simulink model "MultipleAgentsChoice_NoVR"  (Simulink 7.5)
settings: Solver=ode45  StartTime=0.0  StopTime=1000  RelTol=1e-4  AbsTol=1e-4
libraries: simulink x64
(part 4 of 6)

== system MultipleAgentsChoice_NoVR/StatePropagation/SatelliteControlAccel/Agent Body3/Actual Thruster response/Zthruster1 ==
  note: NB:-Agent has no knowledge of red blocks
      |             -Blue blocks prescribed by agent
  note: Tank pressure and thruster selection: must declare number of thrusters
  FeedPressure : Inport  OutDataType=sfix(16)  OutScaling=2^0
  ForceRequest : Inport  Port=2  OutDataType=sfix(16)  OutScaling=2^0
  Data : Inport  Port=3  OutDataType=sfix(16)  OutScaling=2^0
  Reliability : Inport  Port=4  OutDataType=sfix(16)  OutScaling=2^0
  BrokenLine : Inport  Port=5  OutDataType=sfix(16)  OutScaling=2^0
  Bus Creator2 : BusCreator  Inputs=3
  Bus Selector : BusSelector  OutputSignals=ZValves,ZSwitch
  Constant : Constant  OutDataType=sfix(16)  OutScaling=2^0
  Constant1 : Constant  Value=0  OutDataType=sfix(16)  OutScaling=2^0
  Switch : Switch  Criteria=u2 ~= 0
  Thruster1 : Subsystem
  ZData : Outport  OutDataType=sfix(16)  OutScaling=2^0
  Zforces : Outport  Port=2  OutDataType=sfix(16)  OutScaling=2^0
  Activitydata : Outport  Port=3  OutDataType=sfix(16)  OutScaling=2^0
  wires:
  ForceRequest/1 -> Thruster1/4(ForceRequest)  "Zforces"
  Thruster1/1(L1Vent) -> Bus Creator2/1  "L1Vent"
  Thruster1/2(L2Vent) -> Bus Creator2/2  "L2Vent"
  FeedPressure/1 -> Thruster1/2(FeedPressure)
  Constant/1 -> Switch/1
  Constant1/1 -> Switch/3
  Thruster1/4(thrusterData) -> ZData/1  "A3TZ"
  Data/1 -> Bus Selector/1
  Bus Selector/1 -> Thruster1/1(ValveAssign)  "<ZValves>"
  Bus Selector/2 -> Thruster1/3(MainSwitch)  "<ZSwitch>"
  Thruster1/3(Forces) -> Zforces/1, Switch/2
  Switch/1 -> Bus Creator2/3  "Active1"
  Bus Creator2/1 -> Activitydata/1
  Reliability/1 -> Thruster1/5(Reliability)
  BrokenLine/1 -> Thruster1/6(BrokenLine)

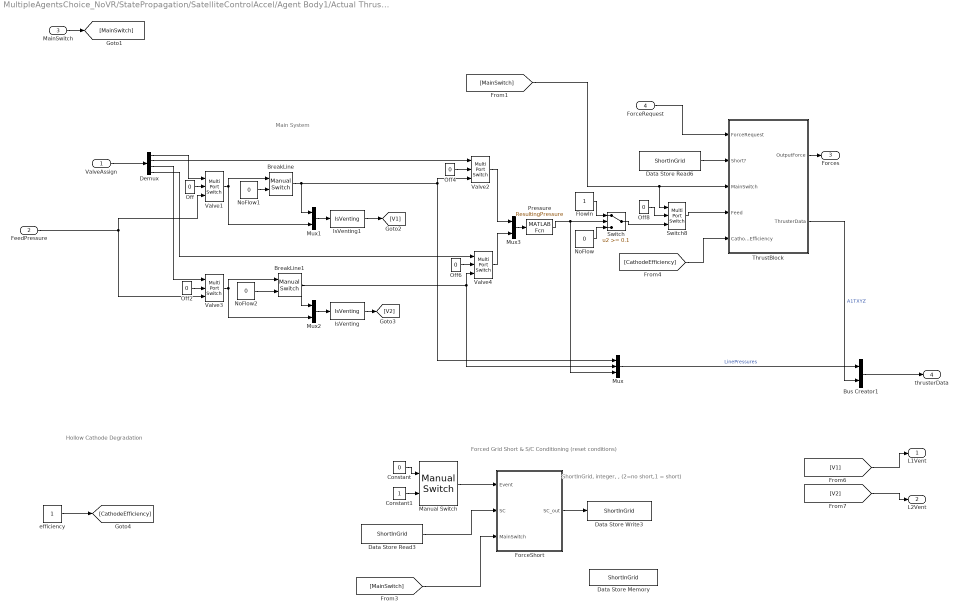
== system MultipleAgentsChoice_NoVR/StatePropagation/SatelliteControlAccel/Agent Body1/Actual Thruster response/XYZthruster/Thruster1 ==
  note: Forced Grid Short & S/C Conditioning (reset conditions)
  note: ShortInGrid, integer, , (2=no short,1 = short)
  note: Hollow Cathode Degradation
  note: Main System
  ValveAssign : Inport  OutDataType=sfix(16)  OutScaling=2^0
  FeedPressure : Inport  Port=2  OutDataType=sfix(16)  OutScaling=2^0
  MainSwitch : Inport  Port=3  OutDataType=sfix(16)  OutScaling=2^0
  ForceRequest : Inport  Port=4  OutDataType=sfix(16)  OutScaling=2^0
  BreakLine : simulink/Signal Routing/Manual Switch  SystemSampleTime=-1  sw=1  action=0  varsize=off
  BreakLine1 : simulink/Signal Routing/Manual Switch  SystemSampleTime=-1  sw=1  action=0  varsize=off
  Bus Creator1 : BusCreator  Inputs=2
  Constant : Constant  Value=0  OutDataType=sfix(16)  OutScaling=2^0
  Constant1 : Constant  OutDataType=sfix(16)  OutScaling=2^0
  Data Store Memory : DataStoreMemory  DataStoreName=ShortInGrid  ReadBeforeWriteMsg=warning  WriteAfterWriteMsg=warning  WriteAfterReadMsg=warning  InitialValue=2  OutDataType=sfix(16)  OutScaling=2^0
  Data Store Read3 : DataStoreRead  DataStoreName=ShortInGrid  SampleTime=0
  Data Store Read6 : DataStoreRead  DataStoreName=ShortInGrid  SampleTime=0
  Data Store Write3 : DataStoreWrite  DataStoreName=ShortInGrid  SampleTime=-1
  Demux : Demux
  FlowIn : Constant  OutDataType=sfix(16)  OutScaling=2^0
  ForceShort : Subsystem
  IsVenting : MATLABFcn  MATLABFcn=IsVenting  OutputDimensions=1
  IsVenting1 : MATLABFcn  MATLABFcn=IsVenting  OutputDimensions=1
  Manual Switch : simulink/Signal Routing/Manual Switch  SystemSampleTime=-1  sw=1  action=0  varsize=off
  Mux : Mux  Inputs=3
  Mux1 : Mux  Inputs=2
  Mux2 : Mux  Inputs=2
  Mux3 : Mux  Inputs=2
  NoFlow : Constant  Value=0  OutDataType=sfix(16)  OutScaling=2^0
  NoFlow1 : Constant  Value=0  OutDataType=sfix(16)  OutScaling=2^0
  NoFlow2 : Constant  Value=0  OutDataType=sfix(16)  OutScaling=2^0
  Off{,2,4,6,8} (5 alike) : Constant  Value=0  OutDataType=sfix(16)  OutScaling=2^0
  Pressure : MATLABFcn  MATLABFcn=ResultingPressure
  Switch : Switch  Threshold=0.1
  Switch8 : MultiPortSwitch  Inputs=2  zeroidx=off
  ThrustBlock : Subsystem
  Valve{1..4} (4 alike) : MultiPortSwitch  Inputs=2  zeroidx=off
  efficiency : Constant  OutDataType=sfix(16)  OutScaling=2^0
  L1Vent : Outport  OutDataType=sfix(16)  OutScaling=2^0
  L2Vent : Outport  Port=2  OutDataType=sfix(16)  OutScaling=2^0
  Forces : Outport  Port=3  OutDataType=sfix(16)  OutScaling=2^0
  thrusterData : Outport  Port=4  OutDataType=sfix(16)  OutScaling=2^0
  wires:
  ForceShort/1(SC_out) -> Data Store Write3/1
  Constant/1 -> Manual Switch/1
  Constant1/1 -> Manual Switch/2
  Manual Switch/1 -> ForceShort/1(Event)
  Data Store Read3/1 -> ForceShort/2(SC)
  [MainSwitch] -> ForceShort/3(MainSwitch)
  efficiency/1 -> [CathodeEfficiency]
  Valve1/1 -> BreakLine/1, Mux1/2
  Valve2/1 -> Mux3/1
  Mux3/1 -> Pressure/1
  BreakLine/1 -> Mux1/1, Valve2/3, Mux/1
  FlowIn/1 -> Switch/1
  NoFlow/1 -> Switch/3
  Switch8/1 -> ThrustBlock/4(Feed)
  Data Store Read6/1 -> ThrustBlock/2(Short?)
  ValveAssign/1 -> Demux/1
  Demux/1 -> Valve1/1
  Demux/2 -> Valve2/1
  Demux/3 -> Valve3/1
  Demux/4 -> Valve4/1
  ThrustBlock/2(ThrusterData) -> Bus Creator1/2  "A1TXYZ"
  ThrustBlock/1(OutputForce) -> Forces/1
  NoFlow1/1 -> BreakLine/2
  Off/1 -> Valve1/2
  Off4/1 -> Valve2/2
  Off2/1 -> Valve3/2
  Off6/1 -> Valve4/2
  Off8/1 -> Switch8/2
  Switch/1 -> Switch8/3
  Mux/1 -> Bus Creator1/1  "LinePressures"
  NoFlow2/1 -> BreakLine1/2
  Valve3/1 -> BreakLine1/1, Mux2/2
  BreakLine1/1 -> Mux2/1, Valve4/3, Mux/2
  [CathodeEfficiency] -> ThrustBlock/5(CathodeEfficiency)
  ForceRequest/1 -> ThrustBlock/1(ForceRequest)
  Bus Creator1/1 -> thrusterData/1
  Mux1/1 -> IsVenting1/1
  Mux2/1 -> IsVenting/1
  Pressure/1 -> Switch/2, Mux/3
  IsVenting1/1 -> [V1]
  IsVenting/1 -> [V2]
  FeedPressure/1 -> Valve1/3, Valve3/3
  MainSwitch/1 -> [MainSwitch]
  Valve4/1 -> Mux3/2
  [MainSwitch] -> ThrustBlock/3(MainSwitch), Switch8/1
  [V1] -> L1Vent/1
  [V2] -> L2Vent/1

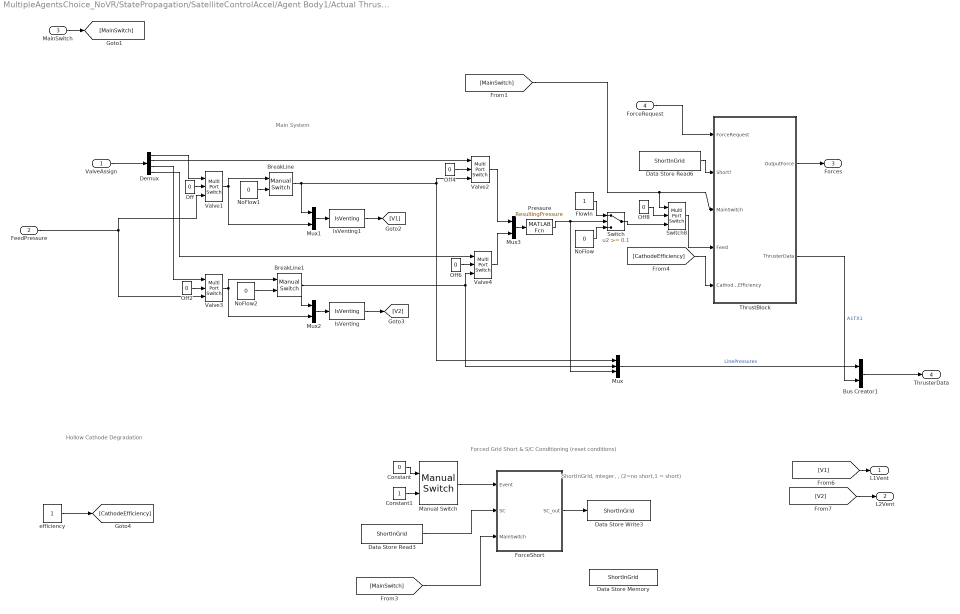
== system MultipleAgentsChoice_NoVR/StatePropagation/SatelliteControlAccel/Agent Body1/Actual Thruster response/Xthruster/Thruster1 ==
  note: Main System
  note: Hollow Cathode Degradation
  note: ShortInGrid, integer, , (2=no short,1 = short)
  note: Forced Grid Short & S/C Conditioning (reset conditions)
  ValveAssign : Inport  OutDataType=sfix(16)  OutScaling=2^0
  FeedPressure : Inport  Port=2  OutDataType=sfix(16)  OutScaling=2^0
  MainSwitch : Inport  Port=3  OutDataType=sfix(16)  OutScaling=2^0
  ForceRequest : Inport  Port=4  OutDataType=sfix(16)  OutScaling=2^0
  BreakLine : simulink/Signal Routing/Manual Switch  SystemSampleTime=-1  sw=1  action=0  varsize=off
  BreakLine1 : simulink/Signal Routing/Manual Switch  SystemSampleTime=-1  sw=1  action=0  varsize=off
  Bus Creator1 : BusCreator  Inputs=2
  Constant : Constant  Value=0  OutDataType=sfix(16)  OutScaling=2^0
  Constant1 : Constant  OutDataType=sfix(16)  OutScaling=2^0
  Data Store Memory : DataStoreMemory  DataStoreName=ShortInGrid  ReadBeforeWriteMsg=warning  WriteAfterWriteMsg=warning  WriteAfterReadMsg=warning  InitialValue=2  OutDataType=sfix(16)  OutScaling=2^0
  Data Store Read3 : DataStoreRead  DataStoreName=ShortInGrid  SampleTime=0
  Data Store Read6 : DataStoreRead  DataStoreName=ShortInGrid  SampleTime=0
  Data Store Write3 : DataStoreWrite  DataStoreName=ShortInGrid  SampleTime=-1
  Demux : Demux
  FlowIn : Constant  OutDataType=sfix(16)  OutScaling=2^0
  ForceShort : Subsystem
  IsVenting : MATLABFcn  MATLABFcn=IsVenting  OutputDimensions=1
  IsVenting1 : MATLABFcn  MATLABFcn=IsVenting  OutputDimensions=1
  Manual Switch : simulink/Signal Routing/Manual Switch  SystemSampleTime=-1  sw=1  action=0  varsize=off
  Mux : Mux  Inputs=3
  Mux1 : Mux  Inputs=2
  Mux2 : Mux  Inputs=2
  Mux3 : Mux  Inputs=2
  NoFlow : Constant  Value=0  OutDataType=sfix(16)  OutScaling=2^0
  NoFlow1 : Constant  Value=0  OutDataType=sfix(16)  OutScaling=2^0
  NoFlow2 : Constant  Value=0  OutDataType=sfix(16)  OutScaling=2^0
  Off{,2,4,6,8} (5 alike) : Constant  Value=0  OutDataType=sfix(16)  OutScaling=2^0
  Pressure : MATLABFcn  MATLABFcn=ResultingPressure
  Switch : Switch  Threshold=0.1
  Switch8 : MultiPortSwitch  Inputs=2  zeroidx=off
  ThrustBlock : Subsystem
  Valve{1..4} (4 alike) : MultiPortSwitch  Inputs=2  zeroidx=off
  efficiency : Constant  OutDataType=sfix(16)  OutScaling=2^0
  L1Vent : Outport  OutDataType=sfix(16)  OutScaling=2^0
  L2Vent : Outport  Port=2  OutDataType=sfix(16)  OutScaling=2^0
  Forces : Outport  Port=3  OutDataType=sfix(16)  OutScaling=2^0
  ThrusterData : Outport  Port=4  OutDataType=sfix(16)  OutScaling=2^0
  wires:
  [MainSwitch] -> Switch8/1, ThrustBlock/3(MainSwitch)
  Valve4/1 -> Mux3/2
  MainSwitch/1 -> [MainSwitch]
  FeedPressure/1 -> Valve3/3, Valve1/3
  IsVenting/1 -> [V2]
  IsVenting1/1 -> [V1]
  Pressure/1 -> Mux/3, Switch/2
  Mux2/1 -> IsVenting/1
  Mux1/1 -> IsVenting1/1
  Bus Creator1/1 -> ThrusterData/1
  ForceRequest/1 -> ThrustBlock/1(ForceRequest)
  [CathodeEfficiency] -> ThrustBlock/5(CathodeEfficiency)
  BreakLine1/1 -> Mux/2, Valve4/3, Mux2/1
  Valve3/1 -> Mux2/2, BreakLine1/1
  NoFlow2/1 -> BreakLine1/2
  Mux/1 -> Bus Creator1/1  "LinePressures"
  Switch/1 -> Switch8/3
  Off8/1 -> Switch8/2
  Off6/1 -> Valve4/2
  Off2/1 -> Valve3/2
  Off4/1 -> Valve2/2
  Off/1 -> Valve1/2
  NoFlow1/1 -> BreakLine/2
  ThrustBlock/1(OutputForce) -> Forces/1
  ThrustBlock/2(ThrusterData) -> Bus Creator1/2  "A1TX1"
  Demux/4 -> Valve4/1
  Demux/3 -> Valve3/1
  Demux/2 -> Valve2/1
  Demux/1 -> Valve1/1
  ValveAssign/1 -> Demux/1
  Data Store Read6/1 -> ThrustBlock/2(Short?)
  Switch8/1 -> ThrustBlock/4(Feed)
  NoFlow/1 -> Switch/3
  FlowIn/1 -> Switch/1
  BreakLine/1 -> Mux/1, Valve2/3, Mux1/1
  Mux3/1 -> Pressure/1
  Valve2/1 -> Mux3/1
  Valve1/1 -> Mux1/2, BreakLine/1
  efficiency/1 -> [CathodeEfficiency]
  [MainSwitch] -> ForceShort/3(MainSwitch)
  Data Store Read3/1 -> ForceShort/2(SC)
  Manual Switch/1 -> ForceShort/1(Event)
  Constant1/1 -> Manual Switch/2
  Constant/1 -> Manual Switch/1
  ForceShort/1(SC_out) -> Data Store Write3/1
  [V1] -> L1Vent/1
  [V2] -> L2Vent/1

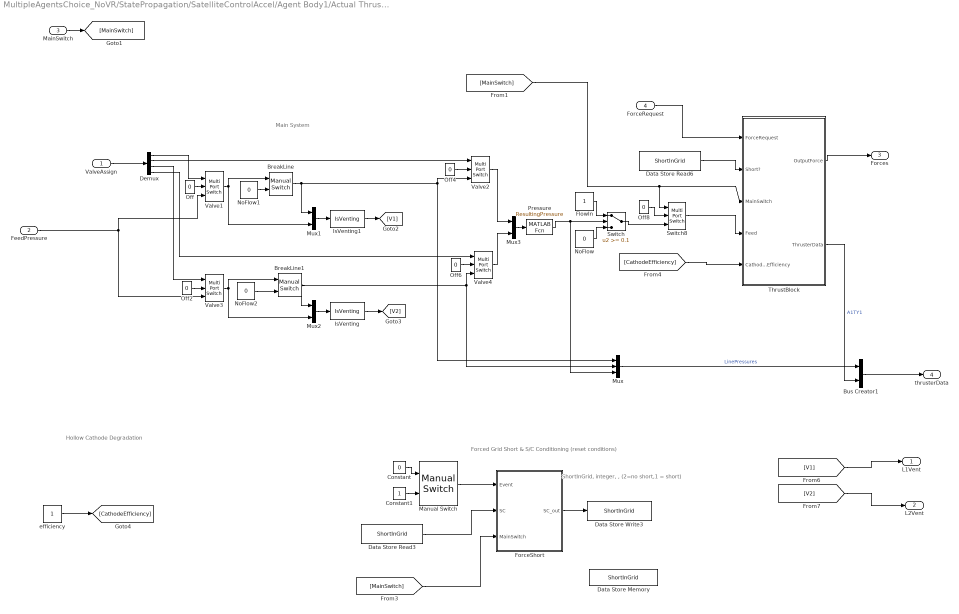
== system MultipleAgentsChoice_NoVR/StatePropagation/SatelliteControlAccel/Agent Body1/Actual Thruster response/Ythruster1/Thruster1 ==
  note: Forced Grid Short & S/C Conditioning (reset conditions)
  note: ShortInGrid, integer, , (2=no short,1 = short)
  note: Hollow Cathode Degradation
  note: Main System
  ValveAssign : Inport  OutDataType=sfix(16)  OutScaling=2^0
  FeedPressure : Inport  Port=2  OutDataType=sfix(16)  OutScaling=2^0
  MainSwitch : Inport  Port=3  OutDataType=sfix(16)  OutScaling=2^0
  ForceRequest : Inport  Port=4  OutDataType=sfix(16)  OutScaling=2^0
  BreakLine : simulink/Signal Routing/Manual Switch  SystemSampleTime=-1  sw=1  action=0  varsize=off
  BreakLine1 : simulink/Signal Routing/Manual Switch  SystemSampleTime=-1  sw=1  action=0  varsize=off
  Bus Creator1 : BusCreator  Inputs=2
  Constant : Constant  Value=0  OutDataType=sfix(16)  OutScaling=2^0
  Constant1 : Constant  OutDataType=sfix(16)  OutScaling=2^0
  Data Store Memory : DataStoreMemory  DataStoreName=ShortInGrid  ReadBeforeWriteMsg=warning  WriteAfterWriteMsg=warning  WriteAfterReadMsg=warning  InitialValue=2  OutDataType=sfix(16)  OutScaling=2^0
  Data Store Read3 : DataStoreRead  DataStoreName=ShortInGrid  SampleTime=0
  Data Store Read6 : DataStoreRead  DataStoreName=ShortInGrid  SampleTime=0
  Data Store Write3 : DataStoreWrite  DataStoreName=ShortInGrid  SampleTime=-1
  Demux : Demux
  FlowIn : Constant  OutDataType=sfix(16)  OutScaling=2^0
  ForceShort : Subsystem
  IsVenting : MATLABFcn  MATLABFcn=IsVenting  OutputDimensions=1
  IsVenting1 : MATLABFcn  MATLABFcn=IsVenting  OutputDimensions=1
  Manual Switch : simulink/Signal Routing/Manual Switch  SystemSampleTime=-1  sw=1  action=0  varsize=off
  Mux : Mux  Inputs=3
  Mux1 : Mux  Inputs=2
  Mux2 : Mux  Inputs=2
  Mux3 : Mux  Inputs=2
  NoFlow : Constant  Value=0  OutDataType=sfix(16)  OutScaling=2^0
  NoFlow1 : Constant  Value=0  OutDataType=sfix(16)  OutScaling=2^0
  NoFlow2 : Constant  Value=0  OutDataType=sfix(16)  OutScaling=2^0
  Off{,2,4,6,8} (5 alike) : Constant  Value=0  OutDataType=sfix(16)  OutScaling=2^0
  Pressure : MATLABFcn  MATLABFcn=ResultingPressure
  Switch : Switch  Threshold=0.1
  Switch8 : MultiPortSwitch  Inputs=2  zeroidx=off
  ThrustBlock : Subsystem
  Valve{1..4} (4 alike) : MultiPortSwitch  Inputs=2  zeroidx=off
  efficiency : Constant  OutDataType=sfix(16)  OutScaling=2^0
  L1Vent : Outport  OutDataType=sfix(16)  OutScaling=2^0
  L2Vent : Outport  Port=2  OutDataType=sfix(16)  OutScaling=2^0
  Forces : Outport  Port=3  OutDataType=sfix(16)  OutScaling=2^0
  thrusterData : Outport  Port=4  OutDataType=sfix(16)  OutScaling=2^0
  wires:
  ForceShort/1(SC_out) -> Data Store Write3/1
  Constant/1 -> Manual Switch/1
  Constant1/1 -> Manual Switch/2
  Manual Switch/1 -> ForceShort/1(Event)
  Data Store Read3/1 -> ForceShort/2(SC)
  [MainSwitch] -> ForceShort/3(MainSwitch)
  efficiency/1 -> [CathodeEfficiency]
  Valve1/1 -> BreakLine/1, Mux1/2
  Valve2/1 -> Mux3/1
  Mux3/1 -> Pressure/1
  BreakLine/1 -> Mux1/1, Valve2/3, Mux/1
  FlowIn/1 -> Switch/1
  NoFlow/1 -> Switch/3
  Switch8/1 -> ThrustBlock/4(Feed)
  Data Store Read6/1 -> ThrustBlock/2(Short?)
  ValveAssign/1 -> Demux/1
  Demux/1 -> Valve1/1
  Demux/2 -> Valve2/1
  Demux/3 -> Valve3/1
  Demux/4 -> Valve4/1
  ThrustBlock/2(ThrusterData) -> Bus Creator1/2  "A1TY1"
  ThrustBlock/1(OutputForce) -> Forces/1
  NoFlow1/1 -> BreakLine/2
  Off/1 -> Valve1/2
  Off4/1 -> Valve2/2
  Off2/1 -> Valve3/2
  Off6/1 -> Valve4/2
  Off8/1 -> Switch8/2
  Switch/1 -> Switch8/3
  Mux/1 -> Bus Creator1/1  "LinePressures"
  NoFlow2/1 -> BreakLine1/2
  Valve3/1 -> BreakLine1/1, Mux2/2
  BreakLine1/1 -> Mux2/1, Valve4/3, Mux/2
  [CathodeEfficiency] -> ThrustBlock/5(CathodeEfficiency)
  ForceRequest/1 -> ThrustBlock/1(ForceRequest)
  Bus Creator1/1 -> thrusterData/1
  Mux1/1 -> IsVenting1/1
  Mux2/1 -> IsVenting/1
  Pressure/1 -> Switch/2, Mux/3
  IsVenting1/1 -> [V1]
  IsVenting/1 -> [V2]
  FeedPressure/1 -> Valve1/3, Valve3/3
  MainSwitch/1 -> [MainSwitch]
  Valve4/1 -> Mux3/2
  [MainSwitch] -> Switch8/1, ThrustBlock/3(MainSwitch)
  [V1] -> L1Vent/1
  [V2] -> L2Vent/1

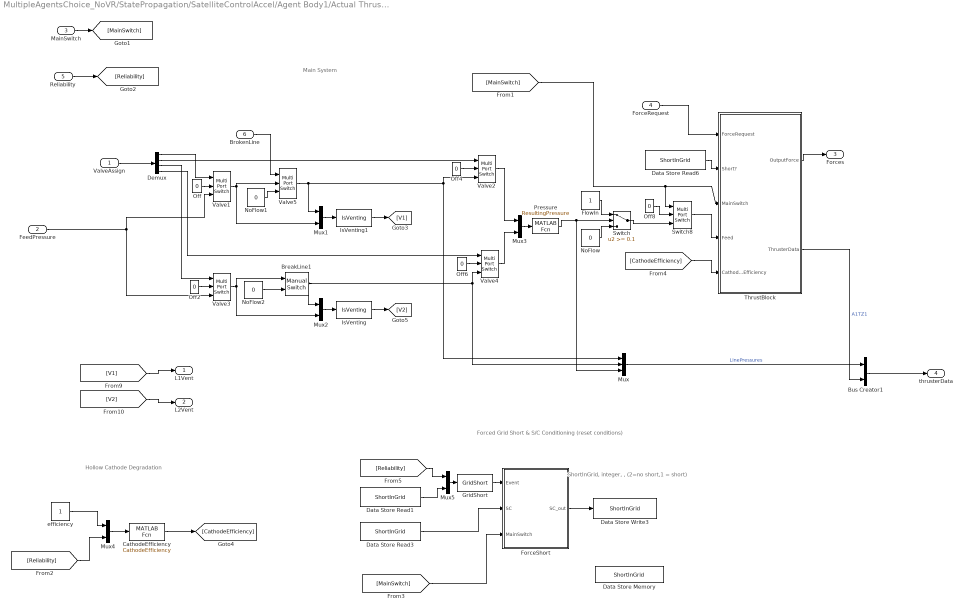
== system MultipleAgentsChoice_NoVR/StatePropagation/SatelliteControlAccel/Agent Body1/Actual Thruster response/Zthruster1/Thruster1 ==
  note: Main System
  note: Hollow Cathode Degradation
  note: ShortInGrid, integer, , (2=no short,1 = short)
  note: Forced Grid Short & S/C Conditioning (reset conditions)
  ValveAssign : Inport  OutDataType=sfix(16)  OutScaling=2^0
  FeedPressure : Inport  Port=2  OutDataType=sfix(16)  OutScaling=2^0
  MainSwitch : Inport  Port=3  OutDataType=sfix(16)  OutScaling=2^0
  ForceRequest : Inport  Port=4  OutDataType=sfix(16)  OutScaling=2^0
  Reliability : Inport  Port=5  OutDataType=sfix(16)  OutScaling=2^0
  BrokenLine : Inport  Port=6  OutDataType=sfix(16)  OutScaling=2^0
  BreakLine1 : simulink/Signal Routing/Manual Switch  SystemSampleTime=-1  sw=1  action=0  varsize=off
  Bus Creator1 : BusCreator  Inputs=2
  CathodeEfficiency : MATLABFcn  MATLABFcn=CathodeEfficiency  OutputDimensions=1
  Data Store Memory : DataStoreMemory  DataStoreName=ShortInGrid  ReadBeforeWriteMsg=warning  WriteAfterWriteMsg=warning  WriteAfterReadMsg=warning  InitialValue=2  OutDataType=sfix(16)  OutScaling=2^0
  Data Store Read1 : DataStoreRead  DataStoreName=ShortInGrid  SampleTime=0
  Data Store Read3 : DataStoreRead  DataStoreName=ShortInGrid  SampleTime=0
  Data Store Read6 : DataStoreRead  DataStoreName=ShortInGrid  SampleTime=0
  Data Store Write3 : DataStoreWrite  DataStoreName=ShortInGrid  SampleTime=-1
  Demux : Demux
  FlowIn : Constant  OutDataType=sfix(16)  OutScaling=2^0
  ForceShort : Subsystem
  GridShort : MATLABFcn  MATLABFcn=GridShort  OutputDimensions=1
  IsVenting : MATLABFcn  MATLABFcn=IsVenting  OutputDimensions=1
  IsVenting1 : MATLABFcn  MATLABFcn=IsVenting  OutputDimensions=1
  Mux : Mux  Inputs=3
  Mux{1..5} (5 alike) : Mux  Inputs=2
  NoFlow : Constant  Value=0  OutDataType=sfix(16)  OutScaling=2^0
  NoFlow1 : Constant  Value=0  OutDataType=sfix(16)  OutScaling=2^0
  NoFlow2 : Constant  Value=0  OutDataType=sfix(16)  OutScaling=2^0
  Off{,2,4,6,8} (5 alike) : Constant  Value=0  OutDataType=sfix(16)  OutScaling=2^0
  Pressure : MATLABFcn  MATLABFcn=ResultingPressure
  Switch : Switch  Threshold=0.1
  Switch8 : MultiPortSwitch  Inputs=2  zeroidx=off
  ThrustBlock : Subsystem
  Valve{1..5} (5 alike) : MultiPortSwitch  Inputs=2  zeroidx=off
  efficiency : Constant  OutDataType=sfix(16)  OutScaling=2^0
  L1Vent : Outport  OutDataType=sfix(16)  OutScaling=2^0
  L2Vent : Outport  Port=2  OutDataType=sfix(16)  OutScaling=2^0
  Forces : Outport  Port=3  OutDataType=sfix(16)  OutScaling=2^0
  thrusterData : Outport  Port=4  OutDataType=sfix(16)  OutScaling=2^0
  wires:
  BrokenLine/1 -> Valve5/1
  [Reliability] -> Mux5/1
  Data Store Read1/1 -> Mux5/2
  Mux5/1 -> GridShort/1
  CathodeEfficiency/1 -> [CathodeEfficiency]
  Mux4/1 -> CathodeEfficiency/1
  [Reliability] -> Mux4/2
  efficiency/1 -> Mux4/1
  Reliability/1 -> [Reliability]
  [MainSwitch] -> Switch8/1, ThrustBlock/3(MainSwitch)
  Valve4/1 -> Mux3/2
  MainSwitch/1 -> [MainSwitch]
  FeedPressure/1 -> Valve3/3, Valve1/3
  IsVenting/1 -> [V2]
  IsVenting1/1 -> [V1]
  Pressure/1 -> Mux/3, Switch/2
  Mux2/1 -> IsVenting/1
  Mux1/1 -> IsVenting1/1
  Bus Creator1/1 -> thrusterData/1
  ForceRequest/1 -> ThrustBlock/1(ForceRequest)
  [CathodeEfficiency] -> ThrustBlock/5(CathodeEfficiency)
  BreakLine1/1 -> Mux/2, Valve4/3, Mux2/1
  Valve3/1 -> Mux2/2, BreakLine1/1
  NoFlow2/1 -> BreakLine1/2
  Mux/1 -> Bus Creator1/1  "LinePressures"
  Switch/1 -> Switch8/3
  Off8/1 -> Switch8/2
  Off6/1 -> Valve4/2
  Off2/1 -> Valve3/2
  Off4/1 -> Valve2/2
  Off/1 -> Valve1/2
  NoFlow1/1 -> Valve5/3
  ThrustBlock/1(OutputForce) -> Forces/1
  ThrustBlock/2(ThrusterData) -> Bus Creator1/2  "A1TZ1"
  Demux/4 -> Valve4/1
  Demux/3 -> Valve3/1
  Demux/2 -> Valve2/1
  Demux/1 -> Valve1/1
  ValveAssign/1 -> Demux/1
  Data Store Read6/1 -> ThrustBlock/2(Short?)
  Switch8/1 -> ThrustBlock/4(Feed)
  NoFlow/1 -> Switch/3
  FlowIn/1 -> Switch/1
  Valve5/1 -> Mux/1, Valve2/3, Mux1/1
  Mux3/1 -> Pressure/1
  Valve2/1 -> Mux3/1
  Valve1/1 -> Mux1/2, Valve5/2
  [MainSwitch] -> ForceShort/3(MainSwitch)
  Data Store Read3/1 -> ForceShort/2(SC)
  GridShort/1 -> ForceShort/1(Event)
  ForceShort/1(SC_out) -> Data Store Write3/1
  [V1] -> L1Vent/1
  [V2] -> L2Vent/1

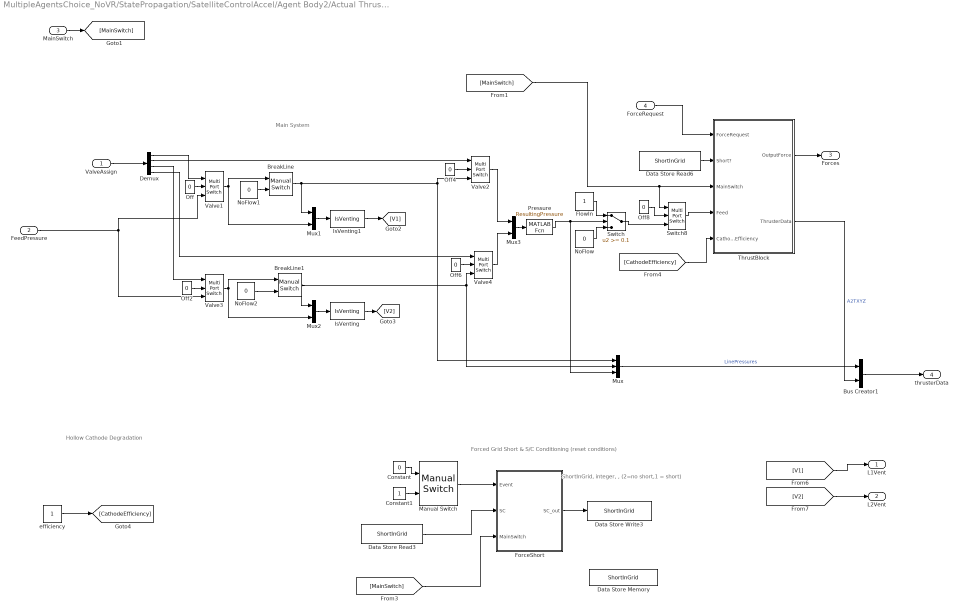
== system MultipleAgentsChoice_NoVR/StatePropagation/SatelliteControlAccel/Agent Body2/Actual Thruster response/XYZthruster/Thruster1 ==
  note: Main System
  note: Hollow Cathode Degradation
  note: ShortInGrid, integer, , (2=no short,1 = short)
  note: Forced Grid Short & S/C Conditioning (reset conditions)
  ValveAssign : Inport  OutDataType=sfix(16)  OutScaling=2^0
  FeedPressure : Inport  Port=2  OutDataType=sfix(16)  OutScaling=2^0
  MainSwitch : Inport  Port=3  OutDataType=sfix(16)  OutScaling=2^0
  ForceRequest : Inport  Port=4  OutDataType=sfix(16)  OutScaling=2^0
  BreakLine : simulink/Signal Routing/Manual Switch  SystemSampleTime=-1  sw=1  action=0  varsize=off
  BreakLine1 : simulink/Signal Routing/Manual Switch  SystemSampleTime=-1  sw=1  action=0  varsize=off
  Bus Creator1 : BusCreator  Inputs=2
  Constant : Constant  Value=0  OutDataType=sfix(16)  OutScaling=2^0
  Constant1 : Constant  OutDataType=sfix(16)  OutScaling=2^0
  Data Store Memory : DataStoreMemory  DataStoreName=ShortInGrid  ReadBeforeWriteMsg=warning  WriteAfterWriteMsg=warning  WriteAfterReadMsg=warning  InitialValue=2  OutDataType=sfix(16)  OutScaling=2^0
  Data Store Read3 : DataStoreRead  DataStoreName=ShortInGrid  SampleTime=0
  Data Store Read6 : DataStoreRead  DataStoreName=ShortInGrid  SampleTime=0
  Data Store Write3 : DataStoreWrite  DataStoreName=ShortInGrid  SampleTime=-1
  Demux : Demux
  FlowIn : Constant  OutDataType=sfix(16)  OutScaling=2^0
  ForceShort : Subsystem
  IsVenting : MATLABFcn  MATLABFcn=IsVenting  OutputDimensions=1
  IsVenting1 : MATLABFcn  MATLABFcn=IsVenting  OutputDimensions=1
  Manual Switch : simulink/Signal Routing/Manual Switch  SystemSampleTime=-1  sw=1  action=0  varsize=off
  Mux : Mux  Inputs=3
  Mux1 : Mux  Inputs=2
  Mux2 : Mux  Inputs=2
  Mux3 : Mux  Inputs=2
  NoFlow : Constant  Value=0  OutDataType=sfix(16)  OutScaling=2^0
  NoFlow1 : Constant  Value=0  OutDataType=sfix(16)  OutScaling=2^0
  NoFlow2 : Constant  Value=0  OutDataType=sfix(16)  OutScaling=2^0
  Off{,2,4,6,8} (5 alike) : Constant  Value=0  OutDataType=sfix(16)  OutScaling=2^0
  Pressure : MATLABFcn  MATLABFcn=ResultingPressure
  Switch : Switch  Threshold=0.1
  Switch8 : MultiPortSwitch  Inputs=2  zeroidx=off
  ThrustBlock : Subsystem
  Valve{1..4} (4 alike) : MultiPortSwitch  Inputs=2  zeroidx=off
  efficiency : Constant  OutDataType=sfix(16)  OutScaling=2^0
  L1Vent : Outport  OutDataType=sfix(16)  OutScaling=2^0
  L2Vent : Outport  Port=2  OutDataType=sfix(16)  OutScaling=2^0
  Forces : Outport  Port=3  OutDataType=sfix(16)  OutScaling=2^0
  thrusterData : Outport  Port=4  OutDataType=sfix(16)  OutScaling=2^0
  wires:
  [MainSwitch] -> Switch8/1, ThrustBlock/3(MainSwitch)
  Valve4/1 -> Mux3/2
  MainSwitch/1 -> [MainSwitch]
  FeedPressure/1 -> Valve3/3, Valve1/3
  IsVenting/1 -> [V2]
  IsVenting1/1 -> [V1]
  Pressure/1 -> Mux/3, Switch/2
  Mux2/1 -> IsVenting/1
  Mux1/1 -> IsVenting1/1
  Bus Creator1/1 -> thrusterData/1
  ForceRequest/1 -> ThrustBlock/1(ForceRequest)
  [CathodeEfficiency] -> ThrustBlock/5(CathodeEfficiency)
  BreakLine1/1 -> Mux/2, Valve4/3, Mux2/1
  Valve3/1 -> Mux2/2, BreakLine1/1
  NoFlow2/1 -> BreakLine1/2
  Mux/1 -> Bus Creator1/1  "LinePressures"
  Switch/1 -> Switch8/3
  Off8/1 -> Switch8/2
  Off6/1 -> Valve4/2
  Off2/1 -> Valve3/2
  Off4/1 -> Valve2/2
  Off/1 -> Valve1/2
  NoFlow1/1 -> BreakLine/2
  ThrustBlock/1(OutputForce) -> Forces/1
  ThrustBlock/2(ThrusterData) -> Bus Creator1/2  "A2TXYZ"
  Demux/4 -> Valve4/1
  Demux/3 -> Valve3/1
  Demux/2 -> Valve2/1
  Demux/1 -> Valve1/1
  ValveAssign/1 -> Demux/1
  Data Store Read6/1 -> ThrustBlock/2(Short?)
  Switch8/1 -> ThrustBlock/4(Feed)
  NoFlow/1 -> Switch/3
  FlowIn/1 -> Switch/1
  BreakLine/1 -> Mux/1, Valve2/3, Mux1/1
  Mux3/1 -> Pressure/1
  Valve2/1 -> Mux3/1
  Valve1/1 -> Mux1/2, BreakLine/1
  efficiency/1 -> [CathodeEfficiency]
  [MainSwitch] -> ForceShort/3(MainSwitch)
  Data Store Read3/1 -> ForceShort/2(SC)
  Manual Switch/1 -> ForceShort/1(Event)
  Constant1/1 -> Manual Switch/2
  Constant/1 -> Manual Switch/1
  ForceShort/1(SC_out) -> Data Store Write3/1
  [V1] -> L1Vent/1
  [V2] -> L2Vent/1

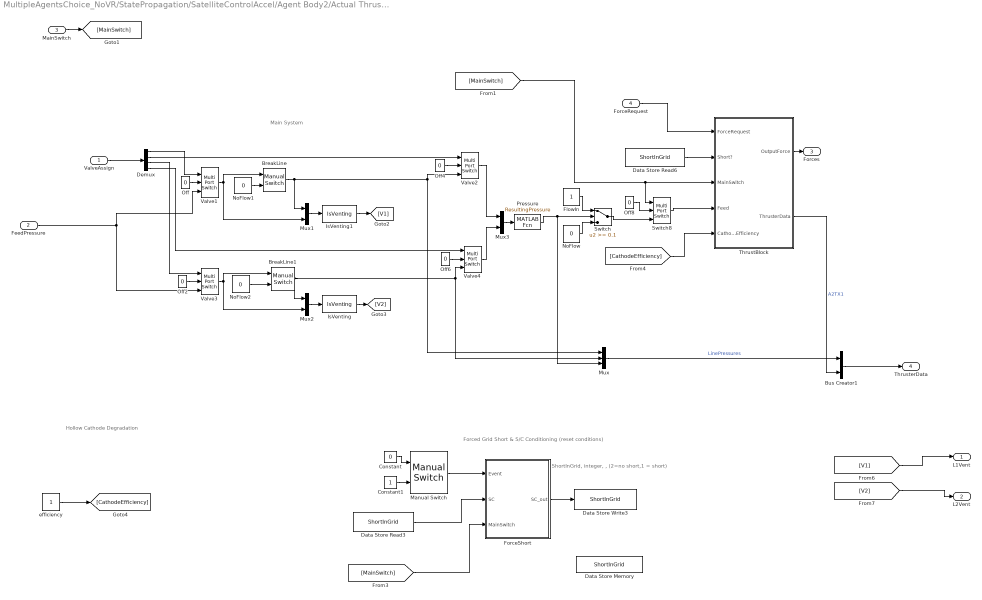
== system MultipleAgentsChoice_NoVR/StatePropagation/SatelliteControlAccel/Agent Body2/Actual Thruster response/Xthruster/Thruster1 ==
  note: Forced Grid Short & S/C Conditioning (reset conditions)
  note: ShortInGrid, integer, , (2=no short,1 = short)
  note: Hollow Cathode Degradation
  note: Main System
  ValveAssign : Inport  OutDataType=sfix(16)  OutScaling=2^0
  FeedPressure : Inport  Port=2  OutDataType=sfix(16)  OutScaling=2^0
  MainSwitch : Inport  Port=3  OutDataType=sfix(16)  OutScaling=2^0
  ForceRequest : Inport  Port=4  OutDataType=sfix(16)  OutScaling=2^0
  BreakLine : simulink/Signal Routing/Manual Switch  SystemSampleTime=-1  sw=1  action=0  varsize=off
  BreakLine1 : simulink/Signal Routing/Manual Switch  SystemSampleTime=-1  sw=1  action=0  varsize=off
  Bus Creator1 : BusCreator  Inputs=2
  Constant : Constant  Value=0  OutDataType=sfix(16)  OutScaling=2^0
  Constant1 : Constant  OutDataType=sfix(16)  OutScaling=2^0
  Data Store Memory : DataStoreMemory  DataStoreName=ShortInGrid  ReadBeforeWriteMsg=warning  WriteAfterWriteMsg=warning  WriteAfterReadMsg=warning  InitialValue=2  OutDataType=sfix(16)  OutScaling=2^0
  Data Store Read3 : DataStoreRead  DataStoreName=ShortInGrid  SampleTime=0
  Data Store Read6 : DataStoreRead  DataStoreName=ShortInGrid  SampleTime=0
  Data Store Write3 : DataStoreWrite  DataStoreName=ShortInGrid  SampleTime=-1
  Demux : Demux
  FlowIn : Constant  OutDataType=sfix(16)  OutScaling=2^0
  ForceShort : Subsystem
  IsVenting : MATLABFcn  MATLABFcn=IsVenting  OutputDimensions=1
  IsVenting1 : MATLABFcn  MATLABFcn=IsVenting  OutputDimensions=1
  Manual Switch : simulink/Signal Routing/Manual Switch  SystemSampleTime=-1  sw=1  action=0  varsize=off
  Mux : Mux  Inputs=3
  Mux1 : Mux  Inputs=2
  Mux2 : Mux  Inputs=2
  Mux3 : Mux  Inputs=2
  NoFlow : Constant  Value=0  OutDataType=sfix(16)  OutScaling=2^0
  NoFlow1 : Constant  Value=0  OutDataType=sfix(16)  OutScaling=2^0
  NoFlow2 : Constant  Value=0  OutDataType=sfix(16)  OutScaling=2^0
  Off{,2,4,6,8} (5 alike) : Constant  Value=0  OutDataType=sfix(16)  OutScaling=2^0
  Pressure : MATLABFcn  MATLABFcn=ResultingPressure
  Switch : Switch  Threshold=0.1
  Switch8 : MultiPortSwitch  Inputs=2  zeroidx=off
  ThrustBlock : Subsystem
  Valve{1..4} (4 alike) : MultiPortSwitch  Inputs=2  zeroidx=off
  efficiency : Constant  OutDataType=sfix(16)  OutScaling=2^0
  L1Vent : Outport  OutDataType=sfix(16)  OutScaling=2^0
  L2Vent : Outport  Port=2  OutDataType=sfix(16)  OutScaling=2^0
  Forces : Outport  Port=3  OutDataType=sfix(16)  OutScaling=2^0
  ThrusterData : Outport  Port=4  OutDataType=sfix(16)  OutScaling=2^0
  wires:
  ForceShort/1(SC_out) -> Data Store Write3/1
  Constant/1 -> Manual Switch/1
  Constant1/1 -> Manual Switch/2
  Manual Switch/1 -> ForceShort/1(Event)
  Data Store Read3/1 -> ForceShort/2(SC)
  [MainSwitch] -> ForceShort/3(MainSwitch)
  efficiency/1 -> [CathodeEfficiency]
  Valve1/1 -> BreakLine/1, Mux1/2
  Valve2/1 -> Mux3/1
  Mux3/1 -> Pressure/1
  BreakLine/1 -> Mux1/1, Valve2/3, Mux/1
  FlowIn/1 -> Switch/1
  NoFlow/1 -> Switch/3
  Switch8/1 -> ThrustBlock/4(Feed)
  Data Store Read6/1 -> ThrustBlock/2(Short?)
  ValveAssign/1 -> Demux/1
  Demux/1 -> Valve1/1
  Demux/2 -> Valve2/1
  Demux/3 -> Valve3/1
  Demux/4 -> Valve4/1
  ThrustBlock/2(ThrusterData) -> Bus Creator1/2  "A2TX1"
  ThrustBlock/1(OutputForce) -> Forces/1
  NoFlow1/1 -> BreakLine/2
  Off/1 -> Valve1/2
  Off4/1 -> Valve2/2
  Off2/1 -> Valve3/2
  Off6/1 -> Valve4/2
  Off8/1 -> Switch8/2
  Switch/1 -> Switch8/3
  Mux/1 -> Bus Creator1/1  "LinePressures"
  NoFlow2/1 -> BreakLine1/2
  Valve3/1 -> BreakLine1/1, Mux2/2
  BreakLine1/1 -> Mux2/1, Valve4/3, Mux/2
  [CathodeEfficiency] -> ThrustBlock/5(CathodeEfficiency)
  ForceRequest/1 -> ThrustBlock/1(ForceRequest)
  Bus Creator1/1 -> ThrusterData/1
  Mux1/1 -> IsVenting1/1
  Mux2/1 -> IsVenting/1
  Pressure/1 -> Switch/2, Mux/3
  IsVenting1/1 -> [V1]
  IsVenting/1 -> [V2]
  FeedPressure/1 -> Valve1/3, Valve3/3
  MainSwitch/1 -> [MainSwitch]
  Valve4/1 -> Mux3/2
  [MainSwitch] -> ThrustBlock/3(MainSwitch), Switch8/1
  [V1] -> L1Vent/1
  [V2] -> L2Vent/1

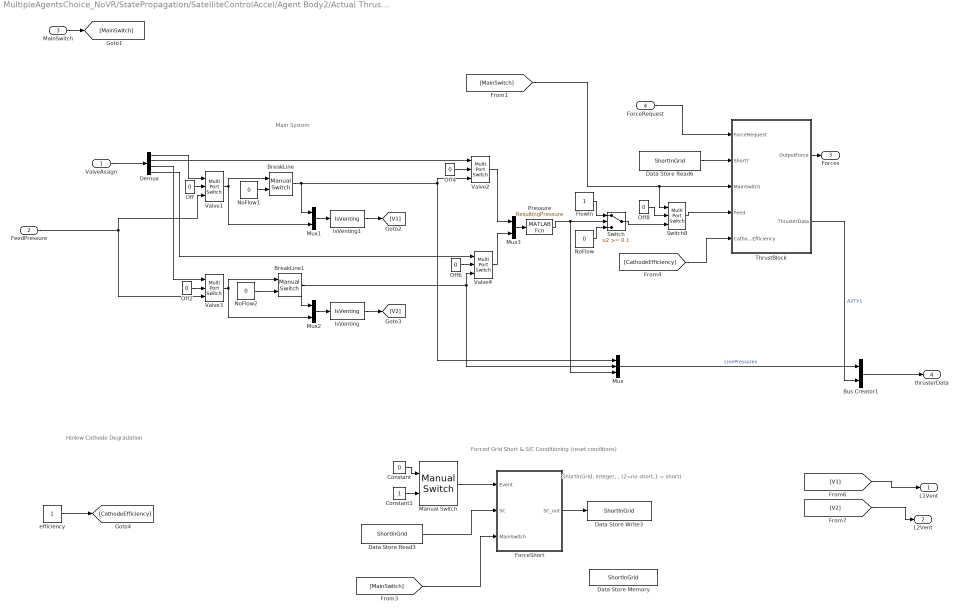
== system MultipleAgentsChoice_NoVR/StatePropagation/SatelliteControlAccel/Agent Body2/Actual Thruster response/Ythruster1/Thruster1 ==
  note: Main System
  note: Hollow Cathode Degradation
  note: ShortInGrid, integer, , (2=no short,1 = short)
  note: Forced Grid Short & S/C Conditioning (reset conditions)
  ValveAssign : Inport  OutDataType=sfix(16)  OutScaling=2^0
  FeedPressure : Inport  Port=2  OutDataType=sfix(16)  OutScaling=2^0
  MainSwitch : Inport  Port=3  OutDataType=sfix(16)  OutScaling=2^0
  ForceRequest : Inport  Port=4  OutDataType=sfix(16)  OutScaling=2^0
  BreakLine : simulink/Signal Routing/Manual Switch  SystemSampleTime=-1  sw=1  action=0  varsize=off
  BreakLine1 : simulink/Signal Routing/Manual Switch  SystemSampleTime=-1  sw=1  action=0  varsize=off
  Bus Creator1 : BusCreator  Inputs=2
  Constant : Constant  Value=0  OutDataType=sfix(16)  OutScaling=2^0
  Constant1 : Constant  OutDataType=sfix(16)  OutScaling=2^0
  Data Store Memory : DataStoreMemory  DataStoreName=ShortInGrid  ReadBeforeWriteMsg=warning  WriteAfterWriteMsg=warning  WriteAfterReadMsg=warning  InitialValue=2  OutDataType=sfix(16)  OutScaling=2^0
  Data Store Read3 : DataStoreRead  DataStoreName=ShortInGrid  SampleTime=0
  Data Store Read6 : DataStoreRead  DataStoreName=ShortInGrid  SampleTime=0
  Data Store Write3 : DataStoreWrite  DataStoreName=ShortInGrid  SampleTime=-1
  Demux : Demux
  FlowIn : Constant  OutDataType=sfix(16)  OutScaling=2^0
  ForceShort : Subsystem
  IsVenting : MATLABFcn  MATLABFcn=IsVenting  OutputDimensions=1
  IsVenting1 : MATLABFcn  MATLABFcn=IsVenting  OutputDimensions=1
  Manual Switch : simulink/Signal Routing/Manual Switch  SystemSampleTime=-1  sw=1  action=0  varsize=off
  Mux : Mux  Inputs=3
  Mux1 : Mux  Inputs=2
  Mux2 : Mux  Inputs=2
  Mux3 : Mux  Inputs=2
  NoFlow : Constant  Value=0  OutDataType=sfix(16)  OutScaling=2^0
  NoFlow1 : Constant  Value=0  OutDataType=sfix(16)  OutScaling=2^0
  NoFlow2 : Constant  Value=0  OutDataType=sfix(16)  OutScaling=2^0
  Off{,2,4,6,8} (5 alike) : Constant  Value=0  OutDataType=sfix(16)  OutScaling=2^0
  Pressure : MATLABFcn  MATLABFcn=ResultingPressure
  Switch : Switch  Threshold=0.1
  Switch8 : MultiPortSwitch  Inputs=2  zeroidx=off
  ThrustBlock : Subsystem
  Valve{1..4} (4 alike) : MultiPortSwitch  Inputs=2  zeroidx=off
  efficiency : Constant  OutDataType=sfix(16)  OutScaling=2^0
  L1Vent : Outport  OutDataType=sfix(16)  OutScaling=2^0
  L2Vent : Outport  Port=2  OutDataType=sfix(16)  OutScaling=2^0
  Forces : Outport  Port=3  OutDataType=sfix(16)  OutScaling=2^0
  thrusterData : Outport  Port=4  OutDataType=sfix(16)  OutScaling=2^0
  wires:
  [MainSwitch] -> ThrustBlock/3(MainSwitch), Switch8/1
  Valve4/1 -> Mux3/2
  MainSwitch/1 -> [MainSwitch]
  FeedPressure/1 -> Valve3/3, Valve1/3
  IsVenting/1 -> [V2]
  IsVenting1/1 -> [V1]
  Pressure/1 -> Mux/3, Switch/2
  Mux2/1 -> IsVenting/1
  Mux1/1 -> IsVenting1/1
  Bus Creator1/1 -> thrusterData/1
  ForceRequest/1 -> ThrustBlock/1(ForceRequest)
  [CathodeEfficiency] -> ThrustBlock/5(CathodeEfficiency)
  BreakLine1/1 -> Mux/2, Valve4/3, Mux2/1
  Valve3/1 -> Mux2/2, BreakLine1/1
  NoFlow2/1 -> BreakLine1/2
  Mux/1 -> Bus Creator1/1  "LinePressures"
  Switch/1 -> Switch8/3
  Off8/1 -> Switch8/2
  Off6/1 -> Valve4/2
  Off2/1 -> Valve3/2
  Off4/1 -> Valve2/2
  Off/1 -> Valve1/2
  NoFlow1/1 -> BreakLine/2
  ThrustBlock/1(OutputForce) -> Forces/1
  ThrustBlock/2(ThrusterData) -> Bus Creator1/2  "A2TY1"
  Demux/4 -> Valve4/1
  Demux/3 -> Valve3/1
  Demux/2 -> Valve2/1
  Demux/1 -> Valve1/1
  ValveAssign/1 -> Demux/1
  Data Store Read6/1 -> ThrustBlock/2(Short?)
  Switch8/1 -> ThrustBlock/4(Feed)
  NoFlow/1 -> Switch/3
  FlowIn/1 -> Switch/1
  BreakLine/1 -> Mux/1, Valve2/3, Mux1/1
  Mux3/1 -> Pressure/1
  Valve2/1 -> Mux3/1
  Valve1/1 -> Mux1/2, BreakLine/1
  efficiency/1 -> [CathodeEfficiency]
  [MainSwitch] -> ForceShort/3(MainSwitch)
  Data Store Read3/1 -> ForceShort/2(SC)
  Manual Switch/1 -> ForceShort/1(Event)
  Constant1/1 -> Manual Switch/2
  Constant/1 -> Manual Switch/1
  ForceShort/1(SC_out) -> Data Store Write3/1
  [V1] -> L1Vent/1
  [V2] -> L2Vent/1

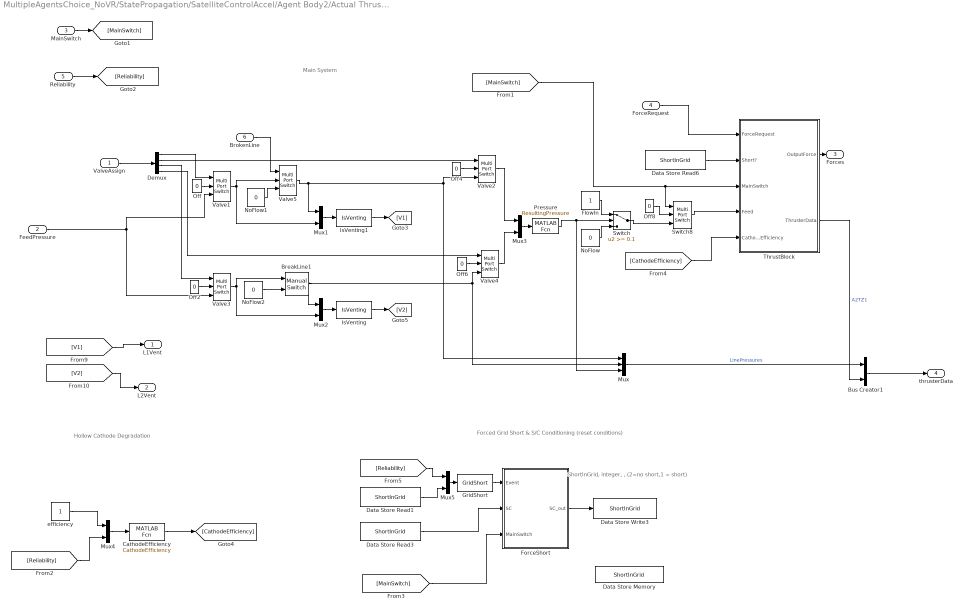
== system MultipleAgentsChoice_NoVR/StatePropagation/SatelliteControlAccel/Agent Body2/Actual Thruster response/Zthruster1/Thruster1 ==
  note: Forced Grid Short & S/C Conditioning (reset conditions)
  note: ShortInGrid, integer, , (2=no short,1 = short)
  note: Hollow Cathode Degradation
  note: Main System
  ValveAssign : Inport  OutDataType=sfix(16)  OutScaling=2^0
  FeedPressure : Inport  Port=2  OutDataType=sfix(16)  OutScaling=2^0
  MainSwitch : Inport  Port=3  OutDataType=sfix(16)  OutScaling=2^0
  ForceRequest : Inport  Port=4  OutDataType=sfix(16)  OutScaling=2^0
  Reliability : Inport  Port=5  OutDataType=sfix(16)  OutScaling=2^0
  BrokenLine : Inport  Port=6  OutDataType=sfix(16)  OutScaling=2^0
  BreakLine1 : simulink/Signal Routing/Manual Switch  SystemSampleTime=-1  sw=1  action=0  varsize=off
  Bus Creator1 : BusCreator  Inputs=2
  CathodeEfficiency : MATLABFcn  MATLABFcn=CathodeEfficiency  OutputDimensions=1
  Data Store Memory : DataStoreMemory  DataStoreName=ShortInGrid  ReadBeforeWriteMsg=warning  WriteAfterWriteMsg=warning  WriteAfterReadMsg=warning  InitialValue=2  OutDataType=sfix(16)  OutScaling=2^0
  Data Store Read1 : DataStoreRead  DataStoreName=ShortInGrid  SampleTime=0
  Data Store Read3 : DataStoreRead  DataStoreName=ShortInGrid  SampleTime=0
  Data Store Read6 : DataStoreRead  DataStoreName=ShortInGrid  SampleTime=0
  Data Store Write3 : DataStoreWrite  DataStoreName=ShortInGrid  SampleTime=-1
  Demux : Demux
  FlowIn : Constant  OutDataType=sfix(16)  OutScaling=2^0
  ForceShort : Subsystem
  GridShort : MATLABFcn  MATLABFcn=GridShort  OutputDimensions=1
  IsVenting : MATLABFcn  MATLABFcn=IsVenting  OutputDimensions=1
  IsVenting1 : MATLABFcn  MATLABFcn=IsVenting  OutputDimensions=1
  Mux : Mux  Inputs=3
  Mux{1..5} (5 alike) : Mux  Inputs=2
  NoFlow : Constant  Value=0  OutDataType=sfix(16)  OutScaling=2^0
  NoFlow1 : Constant  Value=0  OutDataType=sfix(16)  OutScaling=2^0
  NoFlow2 : Constant  Value=0  OutDataType=sfix(16)  OutScaling=2^0
  Off{,2,4,6,8} (5 alike) : Constant  Value=0  OutDataType=sfix(16)  OutScaling=2^0
  Pressure : MATLABFcn  MATLABFcn=ResultingPressure
  Switch : Switch  Threshold=0.1
  Switch8 : MultiPortSwitch  Inputs=2  zeroidx=off
  ThrustBlock : Subsystem
  Valve{1..5} (5 alike) : MultiPortSwitch  Inputs=2  zeroidx=off
  efficiency : Constant  OutDataType=sfix(16)  OutScaling=2^0
  L1Vent : Outport  OutDataType=sfix(16)  OutScaling=2^0
  L2Vent : Outport  Port=2  OutDataType=sfix(16)  OutScaling=2^0
  Forces : Outport  Port=3  OutDataType=sfix(16)  OutScaling=2^0
  thrusterData : Outport  Port=4  OutDataType=sfix(16)  OutScaling=2^0
  wires:
  ForceShort/1(SC_out) -> Data Store Write3/1
  GridShort/1 -> ForceShort/1(Event)
  Data Store Read3/1 -> ForceShort/2(SC)
  [MainSwitch] -> ForceShort/3(MainSwitch)
  Valve1/1 -> Mux1/2, Valve5/2
  Valve2/1 -> Mux3/1
  Mux3/1 -> Pressure/1
  Valve5/1 -> Mux1/1, Valve2/3, Mux/1
  FlowIn/1 -> Switch/1
  NoFlow/1 -> Switch/3
  Switch8/1 -> ThrustBlock/4(Feed)
  Data Store Read6/1 -> ThrustBlock/2(Short?)
  ValveAssign/1 -> Demux/1
  Demux/1 -> Valve1/1
  Demux/2 -> Valve2/1
  Demux/3 -> Valve3/1
  Demux/4 -> Valve4/1
  ThrustBlock/2(ThrusterData) -> Bus Creator1/2  "A2TZ1"
  ThrustBlock/1(OutputForce) -> Forces/1
  NoFlow1/1 -> Valve5/3
  Off/1 -> Valve1/2
  Off4/1 -> Valve2/2
  Off2/1 -> Valve3/2
  Off6/1 -> Valve4/2
  Off8/1 -> Switch8/2
  Switch/1 -> Switch8/3
  Mux/1 -> Bus Creator1/1  "LinePressures"
  NoFlow2/1 -> BreakLine1/2
  Valve3/1 -> BreakLine1/1, Mux2/2
  BreakLine1/1 -> Mux2/1, Valve4/3, Mux/2
  [CathodeEfficiency] -> ThrustBlock/5(CathodeEfficiency)
  ForceRequest/1 -> ThrustBlock/1(ForceRequest)
  Bus Creator1/1 -> thrusterData/1
  Mux1/1 -> IsVenting1/1
  Mux2/1 -> IsVenting/1
  Pressure/1 -> Switch/2, Mux/3
  IsVenting1/1 -> [V1]
  IsVenting/1 -> [V2]
  FeedPressure/1 -> Valve1/3, Valve3/3
  MainSwitch/1 -> [MainSwitch]
  Valve4/1 -> Mux3/2
  [MainSwitch] -> ThrustBlock/3(MainSwitch), Switch8/1
  Reliability/1 -> [Reliability]
  efficiency/1 -> Mux4/1
  [Reliability] -> Mux4/2
  Mux4/1 -> CathodeEfficiency/1
  CathodeEfficiency/1 -> [CathodeEfficiency]
  Mux5/1 -> GridShort/1
  Data Store Read1/1 -> Mux5/2
  [Reliability] -> Mux5/1
  BrokenLine/1 -> Valve5/1
  [V1] -> L1Vent/1
  [V2] -> L2Vent/1

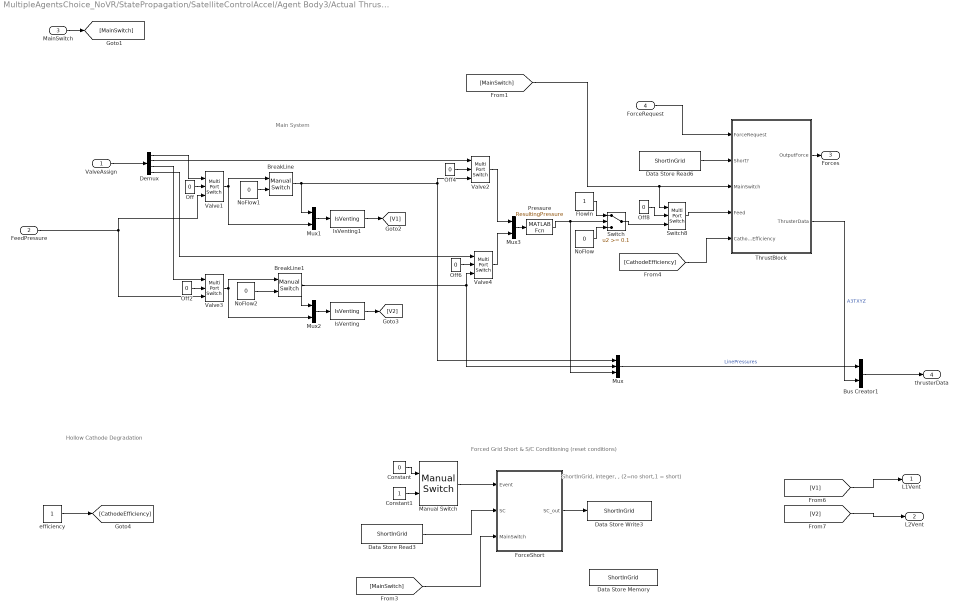
== system MultipleAgentsChoice_NoVR/StatePropagation/SatelliteControlAccel/Agent Body3/Actual Thruster response/XYZthruster/Thruster1 ==
  note: Main System
  note: Hollow Cathode Degradation
  note: ShortInGrid, integer, , (2=no short,1 = short)
  note: Forced Grid Short & S/C Conditioning (reset conditions)
  ValveAssign : Inport  OutDataType=sfix(16)  OutScaling=2^0
  FeedPressure : Inport  Port=2  OutDataType=sfix(16)  OutScaling=2^0
  MainSwitch : Inport  Port=3  OutDataType=sfix(16)  OutScaling=2^0
  ForceRequest : Inport  Port=4  OutDataType=sfix(16)  OutScaling=2^0
  BreakLine : simulink/Signal Routing/Manual Switch  SystemSampleTime=-1  sw=1  action=0  varsize=off
  BreakLine1 : simulink/Signal Routing/Manual Switch  SystemSampleTime=-1  sw=1  action=0  varsize=off
  Bus Creator1 : BusCreator  Inputs=2
  Constant : Constant  Value=0  OutDataType=sfix(16)  OutScaling=2^0
  Constant1 : Constant  OutDataType=sfix(16)  OutScaling=2^0
  Data Store Memory : DataStoreMemory  DataStoreName=ShortInGrid  ReadBeforeWriteMsg=warning  WriteAfterWriteMsg=warning  WriteAfterReadMsg=warning  InitialValue=2  OutDataType=sfix(16)  OutScaling=2^0
  Data Store Read3 : DataStoreRead  DataStoreName=ShortInGrid  SampleTime=0
  Data Store Read6 : DataStoreRead  DataStoreName=ShortInGrid  SampleTime=0
  Data Store Write3 : DataStoreWrite  DataStoreName=ShortInGrid  SampleTime=-1
  Demux : Demux
  FlowIn : Constant  OutDataType=sfix(16)  OutScaling=2^0
  ForceShort : Subsystem
  IsVenting : MATLABFcn  MATLABFcn=IsVenting  OutputDimensions=1
  IsVenting1 : MATLABFcn  MATLABFcn=IsVenting  OutputDimensions=1
  Manual Switch : simulink/Signal Routing/Manual Switch  SystemSampleTime=-1  sw=1  action=0  varsize=off
  Mux : Mux  Inputs=3
  Mux1 : Mux  Inputs=2
  Mux2 : Mux  Inputs=2
  Mux3 : Mux  Inputs=2
  NoFlow : Constant  Value=0  OutDataType=sfix(16)  OutScaling=2^0
  NoFlow1 : Constant  Value=0  OutDataType=sfix(16)  OutScaling=2^0
  NoFlow2 : Constant  Value=0  OutDataType=sfix(16)  OutScaling=2^0
  Off{,2,4,6,8} (5 alike) : Constant  Value=0  OutDataType=sfix(16)  OutScaling=2^0
  Pressure : MATLABFcn  MATLABFcn=ResultingPressure
  Switch : Switch  Threshold=0.1
  Switch8 : MultiPortSwitch  Inputs=2  zeroidx=off
  ThrustBlock : Subsystem
  Valve{1..4} (4 alike) : MultiPortSwitch  Inputs=2  zeroidx=off
  efficiency : Constant  OutDataType=sfix(16)  OutScaling=2^0
  L1Vent : Outport  OutDataType=sfix(16)  OutScaling=2^0
  L2Vent : Outport  Port=2  OutDataType=sfix(16)  OutScaling=2^0
  Forces : Outport  Port=3  OutDataType=sfix(16)  OutScaling=2^0
  thrusterData : Outport  Port=4  OutDataType=sfix(16)  OutScaling=2^0
  wires:
  [MainSwitch] -> Switch8/1, ThrustBlock/3(MainSwitch)
  Valve4/1 -> Mux3/2
  MainSwitch/1 -> [MainSwitch]
  FeedPressure/1 -> Valve3/3, Valve1/3
  IsVenting/1 -> [V2]
  IsVenting1/1 -> [V1]
  Pressure/1 -> Mux/3, Switch/2
  Mux2/1 -> IsVenting/1
  Mux1/1 -> IsVenting1/1
  Bus Creator1/1 -> thrusterData/1
  ForceRequest/1 -> ThrustBlock/1(ForceRequest)
  [CathodeEfficiency] -> ThrustBlock/5(CathodeEfficiency)
  BreakLine1/1 -> Mux/2, Valve4/3, Mux2/1
  Valve3/1 -> Mux2/2, BreakLine1/1
  NoFlow2/1 -> BreakLine1/2
  Mux/1 -> Bus Creator1/1  "LinePressures"
  Switch/1 -> Switch8/3
  Off8/1 -> Switch8/2
  Off6/1 -> Valve4/2
  Off2/1 -> Valve3/2
  Off4/1 -> Valve2/2
  Off/1 -> Valve1/2
  NoFlow1/1 -> BreakLine/2
  ThrustBlock/1(OutputForce) -> Forces/1
  ThrustBlock/2(ThrusterData) -> Bus Creator1/2  "A3TXYZ"
  Demux/4 -> Valve4/1
  Demux/3 -> Valve3/1
  Demux/2 -> Valve2/1
  Demux/1 -> Valve1/1
  ValveAssign/1 -> Demux/1
  Data Store Read6/1 -> ThrustBlock/2(Short?)
  Switch8/1 -> ThrustBlock/4(Feed)
  NoFlow/1 -> Switch/3
  FlowIn/1 -> Switch/1
  BreakLine/1 -> Mux/1, Valve2/3, Mux1/1
  Mux3/1 -> Pressure/1
  Valve2/1 -> Mux3/1
  Valve1/1 -> Mux1/2, BreakLine/1
  efficiency/1 -> [CathodeEfficiency]
  [MainSwitch] -> ForceShort/3(MainSwitch)
  Data Store Read3/1 -> ForceShort/2(SC)
  Manual Switch/1 -> ForceShort/1(Event)
  Constant1/1 -> Manual Switch/2
  Constant/1 -> Manual Switch/1
  ForceShort/1(SC_out) -> Data Store Write3/1
  [V1] -> L1Vent/1
  [V2] -> L2Vent/1

== system MultipleAgentsChoice_NoVR/StatePropagation/SatelliteControlAccel/Agent Body3/Actual Thruster response/Xthruster/Thruster1 ==
  note: Forced Grid Short & S/C Conditioning (reset conditions)
  note: ShortInGrid, integer, , (2=no short,1 = short)
  note: Hollow Cathode Degradation
  note: Main System
  ValveAssign : Inport  OutDataType=sfix(16)  OutScaling=2^0
  FeedPressure : Inport  Port=2  OutDataType=sfix(16)  OutScaling=2^0
  MainSwitch : Inport  Port=3  OutDataType=sfix(16)  OutScaling=2^0
  ForceRequest : Inport  Port=4  OutDataType=sfix(16)  OutScaling=2^0
  BreakLine : simulink/Signal Routing/Manual Switch  SystemSampleTime=-1  sw=1  action=0  varsize=off
  BreakLine1 : simulink/Signal Routing/Manual Switch  SystemSampleTime=-1  sw=1  action=0  varsize=off
  Bus Creator1 : BusCreator  Inputs=2
  Constant : Constant  Value=0  OutDataType=sfix(16)  OutScaling=2^0
  Constant1 : Constant  OutDataType=sfix(16)  OutScaling=2^0
  Data Store Memory : DataStoreMemory  DataStoreName=ShortInGrid  ReadBeforeWriteMsg=warning  WriteAfterWriteMsg=warning  WriteAfterReadMsg=warning  InitialValue=2  OutDataType=sfix(16)  OutScaling=2^0
  Data Store Read3 : DataStoreRead  DataStoreName=ShortInGrid  SampleTime=0
  Data Store Read6 : DataStoreRead  DataStoreName=ShortInGrid  SampleTime=0
  Data Store Write3 : DataStoreWrite  DataStoreName=ShortInGrid  SampleTime=-1
  Demux : Demux
  FlowIn : Constant  OutDataType=sfix(16)  OutScaling=2^0
  ForceShort : Subsystem
  IsVenting : MATLABFcn  MATLABFcn=IsVenting  OutputDimensions=1
  IsVenting1 : MATLABFcn  MATLABFcn=IsVenting  OutputDimensions=1
  Manual Switch : simulink/Signal Routing/Manual Switch  SystemSampleTime=-1  sw=1  action=0  varsize=off
  Mux : Mux  Inputs=3
  Mux1 : Mux  Inputs=2
  Mux2 : Mux  Inputs=2
  Mux3 : Mux  Inputs=2
  NoFlow : Constant  Value=0  OutDataType=sfix(16)  OutScaling=2^0
  NoFlow1 : Constant  Value=0  OutDataType=sfix(16)  OutScaling=2^0
  NoFlow2 : Constant  Value=0  OutDataType=sfix(16)  OutScaling=2^0
  Off{,2,4,6,8} (5 alike) : Constant  Value=0  OutDataType=sfix(16)  OutScaling=2^0
  Pressure : MATLABFcn  MATLABFcn=ResultingPressure
  Switch : Switch  Threshold=0.1
  Switch8 : MultiPortSwitch  Inputs=2  zeroidx=off
  ThrustBlock : Subsystem
  Valve{1..4} (4 alike) : MultiPortSwitch  Inputs=2  zeroidx=off
  efficiency : Constant  OutDataType=sfix(16)  OutScaling=2^0
  L1Vent : Outport  OutDataType=sfix(16)  OutScaling=2^0
  L2Vent : Outport  Port=2  OutDataType=sfix(16)  OutScaling=2^0
  Forces : Outport  Port=3  OutDataType=sfix(16)  OutScaling=2^0
  ThrusterData : Outport  Port=4  OutDataType=sfix(16)  OutScaling=2^0
  wires:
  ForceShort/1(SC_out) -> Data Store Write3/1
  Constant/1 -> Manual Switch/1
  Constant1/1 -> Manual Switch/2
  Manual Switch/1 -> ForceShort/1(Event)
  Data Store Read3/1 -> ForceShort/2(SC)
  [MainSwitch] -> ForceShort/3(MainSwitch)
  efficiency/1 -> [CathodeEfficiency]
  Valve1/1 -> BreakLine/1, Mux1/2
  Valve2/1 -> Mux3/1
  Mux3/1 -> Pressure/1
  BreakLine/1 -> Mux1/1, Valve2/3, Mux/1
  FlowIn/1 -> Switch/1
  NoFlow/1 -> Switch/3
  Switch8/1 -> ThrustBlock/4(Feed)
  Data Store Read6/1 -> ThrustBlock/2(Short?)
  ValveAssign/1 -> Demux/1
  Demux/1 -> Valve1/1
  Demux/2 -> Valve2/1
  Demux/3 -> Valve3/1
  Demux/4 -> Valve4/1
  ThrustBlock/2(ThrusterData) -> Bus Creator1/2  "A3TX1"
  ThrustBlock/1(OutputForce) -> Forces/1
  NoFlow1/1 -> BreakLine/2
  Off/1 -> Valve1/2
  Off4/1 -> Valve2/2
  Off2/1 -> Valve3/2
  Off6/1 -> Valve4/2
  Off8/1 -> Switch8/2
  Switch/1 -> Switch8/3
  Mux/1 -> Bus Creator1/1  "LinePressures"
  NoFlow2/1 -> BreakLine1/2
  Valve3/1 -> BreakLine1/1, Mux2/2
  BreakLine1/1 -> Mux2/1, Valve4/3, Mux/2
  [CathodeEfficiency] -> ThrustBlock/5(CathodeEfficiency)
  ForceRequest/1 -> ThrustBlock/1(ForceRequest)
  Bus Creator1/1 -> ThrusterData/1
  Mux1/1 -> IsVenting1/1
  Mux2/1 -> IsVenting/1
  Pressure/1 -> Switch/2, Mux/3
  IsVenting1/1 -> [V1]
  IsVenting/1 -> [V2]
  FeedPressure/1 -> Valve1/3, Valve3/3
  MainSwitch/1 -> [MainSwitch]
  Valve4/1 -> Mux3/2
  [MainSwitch] -> ThrustBlock/3(MainSwitch), Switch8/1
  [V1] -> L1Vent/1
  [V2] -> L2Vent/1

== system MultipleAgentsChoice_NoVR/StatePropagation/SatelliteControlAccel/Agent Body3/Actual Thruster response/Ythruster1/Thruster1 ==
  note: Main System
  note: Hollow Cathode Degradation
  note: ShortInGrid, integer, , (2=no short,1 = short)
  note: Forced Grid Short & S/C Conditioning (reset conditions)
  ValveAssign : Inport  OutDataType=sfix(16)  OutScaling=2^0
  FeedPressure : Inport  Port=2  OutDataType=sfix(16)  OutScaling=2^0
  MainSwitch : Inport  Port=3  OutDataType=sfix(16)  OutScaling=2^0
  ForceRequest : Inport  Port=4  OutDataType=sfix(16)  OutScaling=2^0
  BreakLine : simulink/Signal Routing/Manual Switch  SystemSampleTime=-1  sw=1  action=0  varsize=off
  BreakLine1 : simulink/Signal Routing/Manual Switch  SystemSampleTime=-1  sw=1  action=0  varsize=off
  Bus Creator1 : BusCreator  Inputs=2
  Constant : Constant  Value=0  OutDataType=sfix(16)  OutScaling=2^0
  Constant1 : Constant  OutDataType=sfix(16)  OutScaling=2^0
  Data Store Memory : DataStoreMemory  DataStoreName=ShortInGrid  ReadBeforeWriteMsg=warning  WriteAfterWriteMsg=warning  WriteAfterReadMsg=warning  InitialValue=2  OutDataType=sfix(16)  OutScaling=2^0
  Data Store Read3 : DataStoreRead  DataStoreName=ShortInGrid  SampleTime=0
  Data Store Read6 : DataStoreRead  DataStoreName=ShortInGrid  SampleTime=0
  Data Store Write3 : DataStoreWrite  DataStoreName=ShortInGrid  SampleTime=-1
  Demux : Demux
  FlowIn : Constant  OutDataType=sfix(16)  OutScaling=2^0
  ForceShort : Subsystem
  IsVenting : MATLABFcn  MATLABFcn=IsVenting  OutputDimensions=1
  IsVenting1 : MATLABFcn  MATLABFcn=IsVenting  OutputDimensions=1
  Manual Switch : simulink/Signal Routing/Manual Switch  SystemSampleTime=-1  sw=1  action=0  varsize=off
  Mux : Mux  Inputs=3
  Mux1 : Mux  Inputs=2
  Mux2 : Mux  Inputs=2
  Mux3 : Mux  Inputs=2
  NoFlow : Constant  Value=0  OutDataType=sfix(16)  OutScaling=2^0
  NoFlow1 : Constant  Value=0  OutDataType=sfix(16)  OutScaling=2^0
  NoFlow2 : Constant  Value=0  OutDataType=sfix(16)  OutScaling=2^0
  Off{,2,4,6,8} (5 alike) : Constant  Value=0  OutDataType=sfix(16)  OutScaling=2^0
  Pressure : MATLABFcn  MATLABFcn=ResultingPressure
  Switch : Switch  Threshold=0.1
  Switch8 : MultiPortSwitch  Inputs=2  zeroidx=off
  ThrustBlock : Subsystem
  Valve{1..4} (4 alike) : MultiPortSwitch  Inputs=2  zeroidx=off
  efficiency : Constant  OutDataType=sfix(16)  OutScaling=2^0
  L1Vent : Outport  OutDataType=sfix(16)  OutScaling=2^0
  L2Vent : Outport  Port=2  OutDataType=sfix(16)  OutScaling=2^0
  Forces : Outport  Port=3  OutDataType=sfix(16)  OutScaling=2^0
  thrusterData : Outport  Port=4  OutDataType=sfix(16)  OutScaling=2^0
  wires:
  [MainSwitch] -> ThrustBlock/3(MainSwitch), Switch8/1
  Valve4/1 -> Mux3/2
  MainSwitch/1 -> [MainSwitch]
  FeedPressure/1 -> Valve3/3, Valve1/3
  IsVenting/1 -> [V2]
  IsVenting1/1 -> [V1]
  Pressure/1 -> Mux/3, Switch/2
  Mux2/1 -> IsVenting/1
  Mux1/1 -> IsVenting1/1
  Bus Creator1/1 -> thrusterData/1
  ForceRequest/1 -> ThrustBlock/1(ForceRequest)
  [CathodeEfficiency] -> ThrustBlock/5(CathodeEfficiency)
  BreakLine1/1 -> Mux/2, Valve4/3, Mux2/1
  Valve3/1 -> Mux2/2, BreakLine1/1
  NoFlow2/1 -> BreakLine1/2
  Mux/1 -> Bus Creator1/1  "LinePressures"
  Switch/1 -> Switch8/3
  Off8/1 -> Switch8/2
  Off6/1 -> Valve4/2
  Off2/1 -> Valve3/2
  Off4/1 -> Valve2/2
  Off/1 -> Valve1/2
  NoFlow1/1 -> BreakLine/2
  ThrustBlock/1(OutputForce) -> Forces/1
  ThrustBlock/2(ThrusterData) -> Bus Creator1/2  "A3TY1"
  Demux/4 -> Valve4/1
  Demux/3 -> Valve3/1
  Demux/2 -> Valve2/1
  Demux/1 -> Valve1/1
  ValveAssign/1 -> Demux/1
  Data Store Read6/1 -> ThrustBlock/2(Short?)
  Switch8/1 -> ThrustBlock/4(Feed)
  NoFlow/1 -> Switch/3
  FlowIn/1 -> Switch/1
  BreakLine/1 -> Mux/1, Valve2/3, Mux1/1
  Mux3/1 -> Pressure/1
  Valve2/1 -> Mux3/1
  Valve1/1 -> Mux1/2, BreakLine/1
  efficiency/1 -> [CathodeEfficiency]
  [MainSwitch] -> ForceShort/3(MainSwitch)
  Data Store Read3/1 -> ForceShort/2(SC)
  Manual Switch/1 -> ForceShort/1(Event)
  Constant1/1 -> Manual Switch/2
  Constant/1 -> Manual Switch/1
  ForceShort/1(SC_out) -> Data Store Write3/1
  [V1] -> L1Vent/1
  [V2] -> L2Vent/1
